simulink model "sonido2"  (R2017a)
settings: Solver=VariableStepAuto  StartTime=0.0  StopTime=10.0  RelTol=1e-3
libraries: dspsrcs4 x4, dspvision x1
settings Model: Creator=Oscar  LastModifiedBy=Oscar

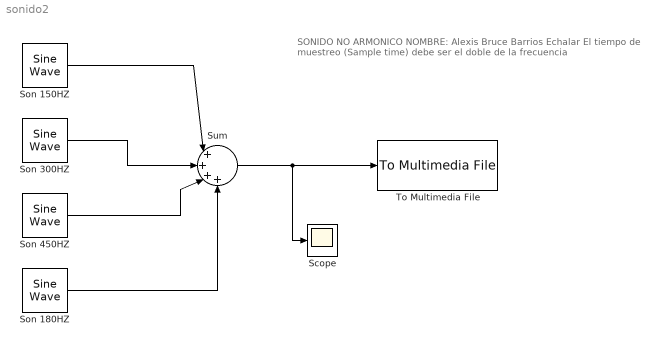
== system sonido2 ==
  note: SONIDO NO ARMONICO
      | NOMBRE: Alexis Bruce Barrios Echalar
      | El tiempo de muestreo (Sample time) debe ser el doble de la frecuencia
  Scope : Scope
  Son 150HZ : dspsrcs4/Sine Wave  Amplitude=0.85  Frequency=150*2  Phase=0  SampleMode=Discrete  OutComplex=Real  CompMethod=Trigonometric fcn  TableSize=Speed  SampleTime=1/1000  SamplesPerFrame=1  ResetState=Restart at time zero  OutputFrames=off  dataType=double  wordLen=16  udDataType=sfix(16)  fracBitsMode=Best precision  numFracBits=15  OutDataTypeStr=double  LastOutDataTypeStr=double
  Son 180HZ : dspsrcs4/Sine Wave  Amplitude=0.85  Frequency=360*2  Phase=0  SampleMode=Discrete  OutComplex=Real  CompMethod=Trigonometric fcn  TableSize=Speed  SampleTime=1/8000  SamplesPerFrame=1  ResetState=Restart at time zero  OutputFrames=off  dataType=double  wordLen=16  udDataType=sfix(16)  fracBitsMode=Best precision  numFracBits=15  OutDataTypeStr=double  LastOutDataTypeStr=double
  Son 300HZ : dspsrcs4/Sine Wave  Amplitude=0.85  Frequency=300*2  Phase=0  SampleMode=Discrete  OutComplex=Real  CompMethod=Trigonometric fcn  TableSize=Speed  SampleTime=1/1000  SamplesPerFrame=1  ResetState=Restart at time zero  OutputFrames=off  dataType=double  wordLen=16  udDataType=sfix(16)  fracBitsMode=Best precision  numFracBits=15  OutDataTypeStr=double  LastOutDataTypeStr=double
  Son 450HZ : dspsrcs4/Sine Wave  Amplitude=0.85  Frequency=450*2  Phase=0  SampleMode=Discrete  OutComplex=Real  CompMethod=Trigonometric fcn  TableSize=Speed  SampleTime=1/8000  SamplesPerFrame=1  ResetState=Restart at time zero  OutputFrames=off  dataType=double  wordLen=16  udDataType=sfix(16)  fracBitsMode=Best precision  numFracBits=15  OutDataTypeStr=double  LastOutDataTypeStr=double
  Sum : Sum  Inputs=|++++
  To Multimedia File : dspvision/To Multimedia File  outputFilename=F:\ALEXIS2\sistemas de control\archivos m\armonia\noarmonico.wav  streamSelection=Audio only  videoCompressor=None (uncompressed)  audioCompressor=None (uncompressed)  imagePorts=Separate color signals  fileType=WAV  audioDatatype=16-bit integer  fourcc=RGB  videoQuality=75  mj2000CompFactor=10
      settings: SourceProductName=Computer Vision System Toolbox  SourceProductBaseCode=VP
  wires:
  Son 150HZ/1 -> Sum/1
  Sum/1 -> To Multimedia File/1, Scope/1
  Son 300HZ/1 -> Sum/2
  Son 450HZ/1 -> Sum/3
  Son 180HZ/1 -> Sum/4
